simulink model "W2P3"  (R2020b)
settings: Solver=VariableStepAuto  StartTime=0.0  StopTime=10.0  RelTol=1e-3
undefined symbols (not defined in the file or in its folder): b, m
settings Model: Creator=saadh  LastModifiedBy=saadh

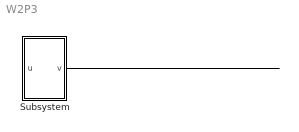
== system W2P3 ==
  Subsystem : Subsystem
  wires:
  Subsystem/1(v) -> ?

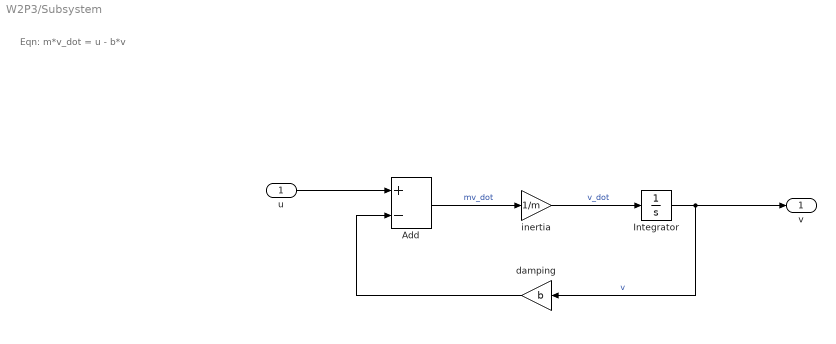
== system W2P3/Subsystem ==
  note: Eqn:
      | m*v_dot = u - b*v
  u : Inport
  Add : Sum  Inputs=+-
  Integrator : Integrator
  damping : Gain  Gain=b
  inertia : Gain  Gain=1/m
  v : Outport
  wires:
  u/1 -> Add/1
  Integrator/1 -> v/1, damping/1  "v"
  damping/1 -> Add/2
  Add/1 -> inertia/1  "mv_dot"
  inertia/1 -> Integrator/1  "v_dot"
